simulink model "six_rod_tensegrity_model_2021a"  (R2021a)
settings: Solver=ode45  StartTime=0  StopTime=Inf  RelTol=1e-1
values from neighbouring files (symbols this model uses):
  grivity_z = -9.80665    [code_for_6_rods_tensegrity.m]
  i = 19    [drive_params.m]
  Jsum = Jd + Jp + Jnagr    (= 9.27e-08)    [drive_params.m]
  km = 9.32 / 1000    (= 0.00932)    [drive_params.m]
  kpdr = 0.81    [drive_params.m]
  kw = 60 / (2*pi * 1020)    (= 0.00936205547599)    [drive_params.m]
  L = 0.14 / 1000    (= 0.00014)    [drive_params.m]
  load_mass = 0.5    [code_for_6_rods_tensegrity.m]
  plane_offset = -(rod_length/2 + 0.032 + rod_radius)    [code_for_6_rods_tensegrity.m]
  R = 5.3    [drive_params.m]
  rod_end_drive_offset = spool_active_length    (= 0.015)    [code_for_6_rods_tensegrity.m]
  rod_end_mass = 0.05    [code_for_6_rods_tensegrity.m]
  rod_end_mass_with_drive = 0.2    [code_for_6_rods_tensegrity.m]
  rod_mass = 0.028    [code_for_6_rods_tensegrity.m]
  rod_mass_with_drive = 0.038    [code_for_6_rods_tensegrity.m]
  rod_radius = 0.004    [code_for_6_rods_tensegrity.m]
undefined symbols (not defined in the file or in its folder): Left_end_cap_1_1, Left_end_cap_2_3, Left_end_cap_3_5, Left_end_cap_4_7, Left_end_cap_5_9, Left_end_cap_6_11, Right_end_cap_1_2, Right_end_cap_2_4, Right_end_cap_3_6, Right_end_cap_4_8, Right_end_cap_5_10, Right_end_cap_6_12, Rod_center_1, Rod_center_2, Rod_center_3, Rod_center_4, Rod_center_5, Rod_center_6, sigbuilder_block, X, Y, Z
libraries: sm_lib x403, nesl_utility x73
(part 4 of 5)

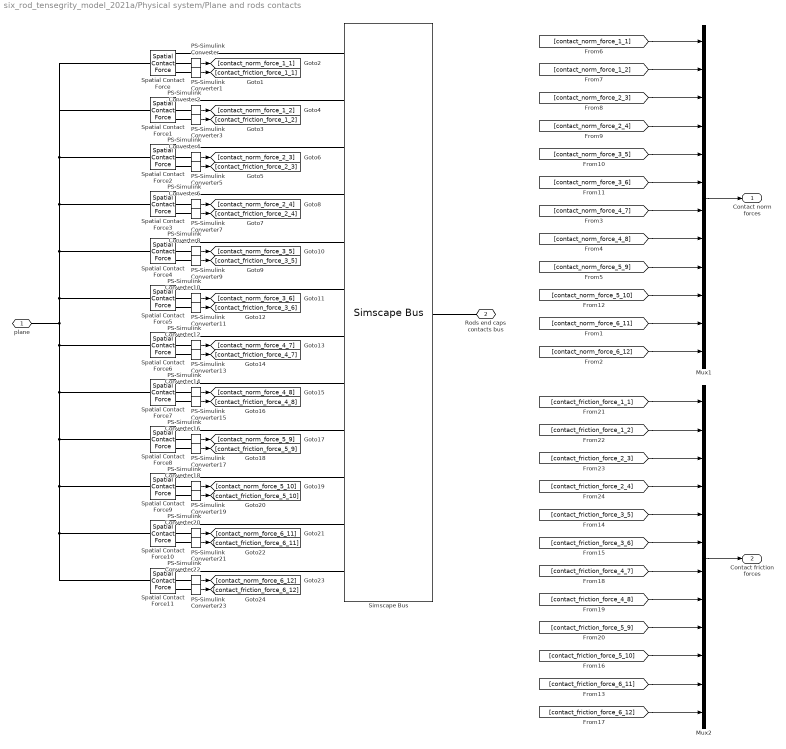
== system six_rod_tensegrity_model_2021a/Physical system/Plane and rods contacts ==
  Mux1 : Mux  Inputs=12
  Mux2 : Mux  Inputs=12
  PS-Simulink Converter{,1..23} (24 alike) : nesl_utility/PS-Simulink Converter  PhysicalDomain=network_engine_domain  SubClassName=ps_output  LeftPortType=input  RightPortType=output  PseudoPeriodic=off  Frequencies=[]  Unit=N  AffineConversion=off
      settings: SourceProductBaseCode=PW,SS
  Simscape Bus : SimscapeBus  HierarchyStrings=Left_end_cap_contact_1_1;Right_end_cap_contact_1_2;Left_end_cap_contact_2_3;Right_end_cap_contact_2_4;Left_end_cap_contact_3_5;Right_end_cap_contact_3_6;Left_end_cap_contact_4_7;Right_end_cap_contact_4_8;Left_end_cap_contact_5_9;Right_end_cap_contact_5_10;Left_end_cap_contact_6_11;Right_end_cap_contact_6_12
  Spatial Contact Force{,1..11} (12 alike) : sm_lib/Forces and Torques/Spatial Contact Force  CoefficientOfDynamicFriction=contact_dynamic_friction_coef  CoefficientOfStaticFriction=contact_static_friction_coef  SenseContactBaseRotation=off  SenseContactBaseTranslation=off  NormalDamping=contact_damping  NormalDampingUnits=N/(m/s)  SenseContactFollowerRotation=off  SenseContactFollowerTranslation=off  SenseContactSignal=off  NormalStiffness=contact_stiffness  NormalStiffnessUnits=N/m  FrictionalCriticalVelocity=contact_critical_velocity  FrictionalCriticalVelocityUnits=m/s  ZeroCrossDetectContactStartAndEnd=off  FrictionType=SmoothStickSlip  SenseFrictionalForceMagnitude=on  SenseNormalForceMagnitude=on  NormalForceType=SmoothSpringDamper  SenseNormalVelocity=off  SenseSeparationDistance=off  SenseTangentialVelocity=off  SenseTangentialVelocityMagnitude=off  NormalTransitionRegionWidth=contact_transition_region_width  NormalTransitionRegionWidthUnits=m
  plane : PMIOPort  Side=Left
  Rods end caps contacts bus : PMIOPort  Port=2  Side=Right
  Contact norm forces : Outport
  Contact friction forces : Outport  Port=2
  wires:
  PS-Simulink Converter/1 -> [contact_norm_force_1_1]
  PS-Simulink Converter1/1 -> [contact_friction_force_1_1]
  PS-Simulink Converter2/1 -> [contact_norm_force_1_2]
  PS-Simulink Converter3/1 -> [contact_friction_force_1_2]
  PS-Simulink Converter5/1 -> [contact_friction_force_2_3]
  PS-Simulink Converter4/1 -> [contact_norm_force_2_3]
  PS-Simulink Converter6/1 -> [contact_norm_force_2_4]
  PS-Simulink Converter7/1 -> [contact_friction_force_2_4]
  PS-Simulink Converter9/1 -> [contact_friction_force_3_5]
  PS-Simulink Converter8/1 -> [contact_norm_force_3_5]
  PS-Simulink Converter10/1 -> [contact_norm_force_3_6]
  PS-Simulink Converter11/1 -> [contact_friction_force_3_6]
  PS-Simulink Converter13/1 -> [contact_friction_force_4_7]
  PS-Simulink Converter12/1 -> [contact_norm_force_4_7]
  PS-Simulink Converter14/1 -> [contact_norm_force_4_8]
  PS-Simulink Converter15/1 -> [contact_friction_force_4_8]
  PS-Simulink Converter17/1 -> [contact_friction_force_5_9]
  PS-Simulink Converter16/1 -> [contact_norm_force_5_9]
  PS-Simulink Converter18/1 -> [contact_norm_force_5_10]
  PS-Simulink Converter19/1 -> [contact_friction_force_5_10]
  PS-Simulink Converter21/1 -> [contact_friction_force_6_11]
  PS-Simulink Converter20/1 -> [contact_norm_force_6_11]
  PS-Simulink Converter22/1 -> [contact_norm_force_6_12]
  PS-Simulink Converter23/1 -> [contact_friction_force_6_12]
  [contact_norm_force_1_1] -> Mux1/1
  [contact_norm_force_2_3] -> Mux1/3
  [contact_norm_force_3_6] -> Mux1/6
  [contact_norm_force_2_4] -> Mux1/4
  Mux1/1 -> Contact norm forces/1
  [contact_norm_force_1_2] -> Mux1/2
  [contact_norm_force_3_5] -> Mux1/5
  [contact_norm_force_4_7] -> Mux1/7
  [contact_norm_force_4_8] -> Mux1/8
  [contact_norm_force_5_9] -> Mux1/9
  [contact_norm_force_5_10] -> Mux1/10
  [contact_norm_force_6_11] -> Mux1/11
  [contact_norm_force_6_12] -> Mux1/12
  [contact_friction_force_6_12] -> Mux2/12
  [contact_friction_force_6_11] -> Mux2/11
  [contact_friction_force_5_10] -> Mux2/10
  [contact_friction_force_5_9] -> Mux2/9
  [contact_friction_force_4_8] -> Mux2/8
  [contact_friction_force_4_7] -> Mux2/7
  [contact_friction_force_3_5] -> Mux2/5
  [contact_friction_force_1_2] -> Mux2/2
  Mux2/1 -> Contact friction forces/1
  [contact_friction_force_2_4] -> Mux2/4
  [contact_friction_force_3_6] -> Mux2/6
  [contact_friction_force_2_3] -> Mux2/3
  [contact_friction_force_1_1] -> Mux2/1
  connections:
  Spatial Contact Force1/RConn1 -- Simscape Bus/LConn2
  Spatial Contact Force3/RConn1 -- Simscape Bus/LConn4
  Spatial Contact Force2/RConn1 -- Simscape Bus/LConn3
  Spatial Contact Force4/RConn1 -- Simscape Bus/LConn5
  Spatial Contact Force5/RConn1 -- Simscape Bus/LConn6
  Spatial Contact Force4/LConn1 -- Spatial Contact Force3/LConn1 -- Spatial Contact Force2/LConn1 -- Spatial Contact Force1/LConn1 -- Spatial Contact Force/LConn1 -- Spatial Contact Force5/LConn1 -- plane/RConn1 -- Spatial Contact Force6/LConn1 -- Spatial Contact Force7/LConn1 -- Spatial Contact Force8/LConn1 -- Spatial Contact Force9/LConn1 -- Spatial Contact Force11/LConn1 -- Spatial Contact Force10/LConn1
  Spatial Contact Force6/RConn1 -- Simscape Bus/LConn7
  Spatial Contact Force11/RConn1 -- Simscape Bus/LConn12
  Spatial Contact Force8/RConn1 -- Simscape Bus/LConn9
  Spatial Contact Force7/RConn1 -- Simscape Bus/LConn8
  Spatial Contact Force10/RConn1 -- Simscape Bus/LConn11
  Spatial Contact Force/RConn1 -- Simscape Bus/LConn1
  Spatial Contact Force9/RConn1 -- Simscape Bus/LConn10
  Rods end caps contacts bus/RConn1 -- Simscape Bus/RConn1
  PS-Simulink Converter/LConn1 -- Spatial Contact Force/RConn2
  Spatial Contact Force/RConn3 -- PS-Simulink Converter1/LConn1
  Spatial Contact Force1/RConn2 -- PS-Simulink Converter2/LConn1
  Spatial Contact Force1/RConn3 -- PS-Simulink Converter3/LConn1
  Spatial Contact Force2/RConn3 -- PS-Simulink Converter5/LConn1
  Spatial Contact Force2/RConn2 -- PS-Simulink Converter4/LConn1
  Spatial Contact Force3/RConn2 -- PS-Simulink Converter6/LConn1
  Spatial Contact Force3/RConn3 -- PS-Simulink Converter7/LConn1
  Spatial Contact Force4/RConn2 -- PS-Simulink Converter8/LConn1
  Spatial Contact Force4/RConn3 -- PS-Simulink Converter9/LConn1
  Spatial Contact Force5/RConn3 -- PS-Simulink Converter11/LConn1
  Spatial Contact Force5/RConn2 -- PS-Simulink Converter10/LConn1
  Spatial Contact Force6/RConn3 -- PS-Simulink Converter13/LConn1
  Spatial Contact Force6/RConn2 -- PS-Simulink Converter12/LConn1
  Spatial Contact Force10/RConn2 -- PS-Simulink Converter20/LConn1
  Spatial Contact Force10/RConn3 -- PS-Simulink Converter21/LConn1
  Spatial Contact Force9/RConn3 -- PS-Simulink Converter19/LConn1
  Spatial Contact Force9/RConn2 -- PS-Simulink Converter18/LConn1
  Spatial Contact Force8/RConn3 -- PS-Simulink Converter17/LConn1
  Spatial Contact Force8/RConn2 -- PS-Simulink Converter16/LConn1
  Spatial Contact Force7/RConn3 -- PS-Simulink Converter15/LConn1
  Spatial Contact Force7/RConn2 -- PS-Simulink Converter14/LConn1
  Spatial Contact Force11/RConn3 -- PS-Simulink Converter23/LConn1
  Spatial Contact Force11/RConn2 -- PS-Simulink Converter22/LConn1

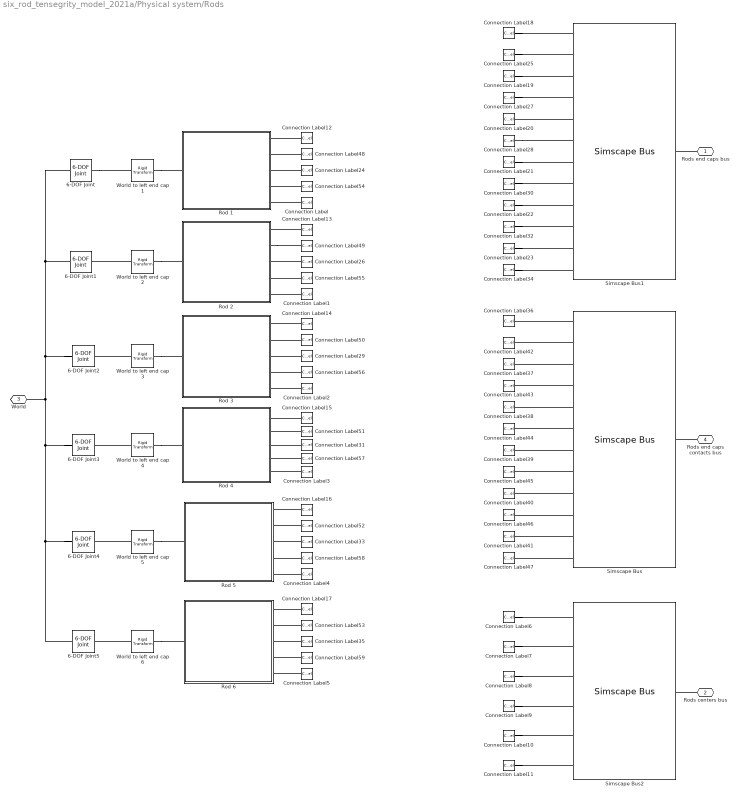
== system six_rod_tensegrity_model_2021a/Physical system/Rods ==
  6-DOF Joint{,1..5} (6 alike) : sm_lib/Joints/6-DOF Joint  JointMode=Normal  SenseConstraintForce=off  SenseConstraintForceX=off  SenseConstraintForceY=off  SenseConstraintForceZ=off  SenseConstraintTorque=off  SenseConstraintTorqueX=off  SenseConstraintTorqueY=off  SenseConstraintTorqueZ=off  SenseTotalForce=off  SenseTotalForceX=off  SenseTotalForceY=off  SenseTotalForceZ=off  SenseTotalTorque=off  SenseTotalTorqueX=off  SenseTotalTorqueY=off  SenseTotalTorqueZ=off  CompositeWrenchDir=FollowerOnBase  CompositeWrenchFrame=BaseFrame  PxEquilibriumPosition=0  PxEquilibriumPositionUnits=m  PxSpringStiffness=0  PxSpringStiffnessUnits=N/m  PxDampingCoefficient=0  PxDampingCoefficientUnits=N/(m/s)  PxTorqueActuationMode=NoTorque  PxMotionActuationMode=ComputedMotion  PxSensePosition=off  PxSenseVelocity=off  PxSenseAcceleration=off  PxSenseTorqueForce=off  PxSenseLowerLimitTorqueForce=off  PxSenseUpperLimitTorqueForce=off  PxLowerLimitSpecify=off  PxLowerLimitBound=-1  PxLowerLimitBoundUnits=m  PxLowerLimitStiffness=1e6  PxLowerLimitStiffnessUnits=N/m  PxLowerLimitDamping=1e3  PxLowerLimitDampingUnits=N/(m/s)  PxLowerLimitTransitionRegionWidth=1e-4  PxLowerLimitTransitionRegionWidthUnits=m  PxUpperLimitSpecify=off  PxUpperLimitBound=1  PxUpperLimitBoundUnits=m  PxUpperLimitStiffness=1e6  PxUpperLimitStiffnessUnits=N/m  PxUpperLimitDamping=1e3  PxUpperLimitDampingUnits=N/(m/s)  PxUpperLimitTransitionRegionWidth=1e-4  PxUpperLimitTransitionRegionWidthUnits=m  PxPositionTargetSpecify=off  PxPositionTargetPriority=High  PxPositionTargetValue=0  PxPositionTargetValueUnits=m  PxVelocityTargetSpecify=off  PxVelocityTargetPriority=High  PxVelocityTargetValue=0  PxVelocityTargetValueUnits=m/s  PyEquilibriumPosition=0  PyEquilibriumPositionUnits=m  PySpringStiffness=0  PySpringStiffnessUnits=N/m  PyDampingCoefficient=0  PyDampingCoefficientUnits=N/(m/s)  PyTorqueActuationMode=NoTorque  PyMotionActuationMode=ComputedMotion  PySensePosition=off  PySenseVelocity=off  PySenseAcceleration=off  PySenseTorqueForce=off  PySenseLowerLimitTorqueForce=off  PySenseUpperLimitTorqueForce=off  PyLowerLimitSpecify=off  PyLowerLimitBound=-1  PyLowerLimitBoundUnits=m  PyLowerLimitStiffness=1e6  PyLowerLimitStiffnessUnits=N/m  PyLowerLimitDamping=1e3  PyLowerLimitDampingUnits=N/(m/s)  PyLowerLimitTransitionRegionWidth=1e-4  PyLowerLimitTransitionRegionWidthUnits=m  PyUpperLimitSpecify=off  PyUpperLimitBound=1  PyUpperLimitBoundUnits=m  PyUpperLimitStiffness=1e6  PyUpperLimitStiffnessUnits=N/m  PyUpperLimitDamping=1e3  PyUpperLimitDampingUnits=N/(m/s)  PyUpperLimitTransitionRegionWidth=1e-4  PyUpperLimitTransitionRegionWidthUnits=m  PyPositionTargetSpecify=off  PyPositionTargetPriority=High  PyPositionTargetValue=0  PyPositionTargetValueUnits=m  PyVelocityTargetSpecify=off  PyVelocityTargetPriority=High  PyVelocityTargetValue=0  PyVelocityTargetValueUnits=m/s  PzEquilibriumPosition=0  PzEquilibriumPositionUnits=m  PzSpringStiffness=0  PzSpringStiffnessUnits=N/m  PzDampingCoefficient=0  PzDampingCoefficientUnits=N/(m/s)  PzTorqueActuationMode=NoTorque  PzMotionActuationMode=ComputedMotion  PzSensePosition=off  PzSenseVelocity=off  PzSenseAcceleration=off  PzSenseTorqueForce=off  PzSenseLowerLimitTorqueForce=off  PzSenseUpperLimitTorqueForce=off  PzLowerLimitSpecify=off  PzLowerLimitBound=-1  PzLowerLimitBoundUnits=m  PzLowerLimitStiffness=1e6  PzLowerLimitStiffnessUnits=N/m  PzLowerLimitDamping=1e3  PzLowerLimitDampingUnits=N/(m/s)  PzLowerLimitTransitionRegionWidth=1e-4  PzLowerLimitTransitionRegionWidthUnits=m  PzUpperLimitSpecify=off  PzUpperLimitBound=1  PzUpperLimitBoundUnits=m  PzUpperLimitStiffness=1e6  PzUpperLimitStiffnessUnits=N/m  PzUpperLimitDamping=1e3  PzUpperLimitDampingUnits=N/(m/s)  PzUpperLimitTransitionRegionWidth=1e-4  PzUpperLimitTransitionRegionWidthUnits=m  PzPositionTargetSpecify=off  PzPositionTargetPriority=High  PzPositionTargetValue=0  PzPositionTargetValueUnits=m  PzVelocityTargetSpecify=off  PzVelocityTargetPriority=High  PzVelocityTargetValue=0  PzVelocityTargetValueUnits=m/s  SphDefPosRotationMethod=None  SphDefPosRotationAngleUnits=deg  SphDefPosRotationStandardAxis=+Z  SphDefPosRotationAngle=0.0  SphDefPosRotationArbitraryAxis=[0 0 1]  SphDefPosFollAlignAxisA=+X  SphDefPosBaseAlignAxisA=+Y  SphDefPosFollAlignAxisB=+Y  SphDefPosBaseAlignAxisB=+Z  SphDefPosRotationSequenceAxes=FollowerAxes  SphDefPosRotationSequence=XYX  SphDefPosRotationSequenceAngles=[0 0 0]  SphDefPosRotationSequenceAnglesUnits=deg  SphDefPosRotationMatrix=[1 0 0; 0 1 0; 0 0 1]  SphEqPosRotationMethod=None  SphEqPosRotationAngleUnits=deg  SphEqPosRotationStandardAxis=+Z  SphEqPosRotationAngle=0.0  SphEqPosRotationArbitraryAxis=[0 0 1]  SphEqPosFollAlignAxisA=+X  SphEqPosBaseAlignAxisA=+Y  SphEqPosFollAlignAxisB=+Y  SphEqPosBaseAlignAxisB=+Z  SphEqPosRotationSequenceAxes=FollowerAxes  SphEqPosRotationSequence=XYX  SphEqPosRotationSequenceAngles=[0 0 0]  SphEqPosRotationSequenceAnglesUnits=deg  SphEqPosRotationMatrix=[1 0 0; 0 1 0; 0 0 1]  SphSpringStiffness=0  SphSpringStiffnessUnits=N*m/deg  SphDampingCoefficient=0  SphDampingCoefficientUnits=N*m/(deg/s)  SphActuateTorqueX=off  SphActuateTorqueY=off  SphActuateTorqueZ=off  SphActuateTorque=off  SphTorqueActuationMode=NoTorque  SphMotionActuationMode=ComputedMotion  SphActuationFrame=BaseFrame  SphSensePosition=off  SphSenseVelocityX=off  SphSenseVelocityY=off  SphSenseVelocityZ=off  SphSenseVelocity=off  SphSenseAccelerationX=off  SphSenseAccelerationY=off  SphSenseAccelerationZ=off  SphSenseAcceleration=off  SphSenseTorqueX=off  SphSenseTorqueY=off  SphSenseTorqueZ=off  SphSenseTorqueForce=off  SphSenseLowerLimitTorqueMag=off  SphSenseUpperLimitTorqueMag=off  SphSensingFrame=BaseFrame  SphLowerLimitSpecify=off  SphLowerLimitBound=15  SphLowerLimitBoundUnits=deg  SphLowerLimitStiffness=1e4  SphLowerLimitStiffnessUnits=N*m/deg  SphLowerLimitDamping=10  SphLowerLimitDampingUnits=N*m/(deg/s)  SphLowerLimitTransitionRegionWidth=0.1  SphLowerLimitTransitionRegionWidthUnits=deg  SphUpperLimitSpecify=off  SphUpperLimitBound=45  SphUpperLimitBoundUnits=deg  SphUpperLimitStiffness=1e4  SphUpperLimitStiffnessUnits=N*m/deg  SphUpperLimitDamping=10  SphUpperLimitDampingUnits=N*m/(deg/s)  SphUpperLimitTransitionRegionWidth=0.1  SphUpperLimitTransitionRegionWidthUnits=deg  SphPositionTargetRotationMethod=None  SphPositionTargetRotationAngleUnits=deg  SphPositionTargetRotationStandardAxis=+Z  SphPositionTargetRotationAngle=0.0  SphPositionTargetRotationArbitraryAxis=[0 0 1]  SphPositionTargetFollAlignAxisA=+X  SphPositionTargetBaseAlignAxisA=+Y  SphPositionTargetFollAlignAxisB=+Y  SphPositionTargetBaseAlignAxisB=+Z  SphPositionTargetRotationSequenceAxes=FollowerAxes  SphPositionTargetRotationSequence=XYX  SphPositionTargetRotationSequenceAngles=[0 0 0]  SphPositionTargetRotationSequenceAnglesUnits=deg  SphPositionTargetRotationMatrix=[1 0 0; 0 1 0; 0 0 1]  SphPositionTargetSpecify=off  SphPositionTargetPriority=High  SphVelocityTargetValue=[0 0 0]  SphVelocityTargetValueUnits=deg/s  SphVelocityTargetSpecify=off  SphVelocityTargetPriority=High  SphVelocityTargetInFollowerFrame=on
  Connection Label : ConnectionLabel  Label=Rod_center_1
  Connection Label1 : ConnectionLabel  Label=Rod_center_2
  Connection Label10 : ConnectionLabel  Label=Rod_center_5
  Connection Label11 : ConnectionLabel  Label=Rod_center_6
  Connection Label12 : ConnectionLabel  Label=Left_end_cap_1_1
  Connection Label13 : ConnectionLabel  Label=Left_end_cap_2_3
  Connection Label14 : ConnectionLabel  Label=Left_end_cap_3_5
  Connection Label15 : ConnectionLabel  Label=Left_end_cap_4_7
  Connection Label16 : ConnectionLabel  Label=Left_end_cap_5_9
  Connection Label17 : ConnectionLabel  Label=Left_end_cap_6_11
  Connection Label18 : ConnectionLabel  Label=Left_end_cap_1_1
  Connection Label19 : ConnectionLabel  Label=Left_end_cap_2_3
  Connection Label2 : ConnectionLabel  Label=Rod_center_3
  Connection Label20 : ConnectionLabel  Label=Left_end_cap_3_5
  Connection Label21 : ConnectionLabel  Label=Left_end_cap_4_7
  Connection Label22 : ConnectionLabel  Label=Left_end_cap_5_9
  Connection Label23 : ConnectionLabel  Label=Left_end_cap_6_11
  Connection Label24 : ConnectionLabel  Label=Right_end_cap_1_2
  Connection Label25 : ConnectionLabel  Label=Right_end_cap_1_2
  Connection Label26 : ConnectionLabel  Label=Right_end_cap_2_4
  Connection Label27 : ConnectionLabel  Label=Right_end_cap_2_4
  Connection Label28 : ConnectionLabel  Label=Right_end_cap_3_6
  Connection Label29 : ConnectionLabel  Label=Right_end_cap_3_6
  Connection Label3 : ConnectionLabel  Label=Rod_center_4
  Connection Label30 : ConnectionLabel  Label=Right_end_cap_4_8
  Connection Label31 : ConnectionLabel  Label=Right_end_cap_4_8
  Connection Label32 : ConnectionLabel  Label=Right_end_cap_5_10
  Connection Label33 : ConnectionLabel  Label=Right_end_cap_5_10
  Connection Label34 : ConnectionLabel  Label=Right_end_cap_6_12
  Connection Label35 : ConnectionLabel  Label=Right_end_cap_6_12
  Connection Label36 : ConnectionLabel  Label=Left_end_cap_contact_1_1
  Connection Label37 : ConnectionLabel  Label=Left_end_cap_contact_2_3
  Connection Label38 : ConnectionLabel  Label=Left_end_cap_contact_3_5
  Connection Label39 : ConnectionLabel  Label=Left_end_cap_contact_4_7
  Connection Label4 : ConnectionLabel  Label=Rod_center_5
  Connection Label40 : ConnectionLabel  Label=Left_end_cap_contact_5_9
  Connection Label41 : ConnectionLabel  Label=Left_end_cap_contact_6_11
  Connection Label42 : ConnectionLabel  Label=Right_end_cap_contact_1_2
  Connection Label43 : ConnectionLabel  Label=Right_end_cap_contact_2_4
  Connection Label44 : ConnectionLabel  Label=Right_end_cap_contact_3_6
  Connection Label45 : ConnectionLabel  Label=Right_end_cap_contact_4_8
  Connection Label46 : ConnectionLabel  Label=Right_end_cap_contact_5_10
  Connection Label47 : ConnectionLabel  Label=Right_end_cap_contact_6_12
  Connection Label48 : ConnectionLabel  Label=Left_end_cap_contact_1_1
  Connection Label49 : ConnectionLabel  Label=Left_end_cap_contact_2_3
  Connection Label5 : ConnectionLabel  Label=Rod_center_6
  Connection Label50 : ConnectionLabel  Label=Left_end_cap_contact_3_5
  Connection Label51 : ConnectionLabel  Label=Left_end_cap_contact_4_7
  Connection Label52 : ConnectionLabel  Label=Left_end_cap_contact_5_9
  Connection Label53 : ConnectionLabel  Label=Left_end_cap_contact_6_11
  Connection Label54 : ConnectionLabel  Label=Right_end_cap_contact_1_2
  Connection Label55 : ConnectionLabel  Label=Right_end_cap_contact_2_4
  Connection Label56 : ConnectionLabel  Label=Right_end_cap_contact_3_6
  Connection Label57 : ConnectionLabel  Label=Right_end_cap_contact_4_8
  Connection Label58 : ConnectionLabel  Label=Right_end_cap_contact_5_10
  Connection Label59 : ConnectionLabel  Label=Right_end_cap_contact_6_12
  Connection Label6 : ConnectionLabel  Label=Rod_center_1
  Connection Label7 : ConnectionLabel  Label=Rod_center_2
  Connection Label8 : ConnectionLabel  Label=Rod_center_3
  Connection Label9 : ConnectionLabel  Label=Rod_center_4
  Rod 1 : Subsystem
      mask Display: image(imread('tensegrity_rod.jpg'))
  Rod 2 : Subsystem
      mask Display: image(imread('tensegrity_rod.jpg'))
  Rod 3 : Subsystem
      mask Display: image(imread('tensegrity_rod.jpg'))
  Rod 4 : Subsystem
      mask Display: image(imread('tensegrity_rod.jpg'))
  Rod 5 : Subsystem
      mask Display: image(imread('tensegrity_rod.jpg'))
  Rod 6 : Subsystem
      mask Display: image(imread('tensegrity_rod.jpg'))
  Simscape Bus : SimscapeBus  HierarchyStrings=Left_end_cap_contact_1_1;Right_end_cap_contact_1_2;Left_end_cap_contact_2_3;Right_end_cap_contact_2_4;Left_end_cap_contact_3_5;Right_end_cap_contact_3_6;Left_end_cap_contact_4_7;Right_end_cap_contact_4_8;Left_end_cap_contact_5_9;Right_end_cap_contact_5_10;Left_end_cap_contact_6_11;Right_end_cap_contact_6_12
  Simscape Bus1 : SimscapeBus  HierarchyStrings=Left_end_cap_1_1;Right_end_cap_1_2;Left_end_cap_2_3;Right_end_cap_2_4;Left_end_cap_3_5;Right_end_cap_3_6;Left_end_cap_4_7;Right_end_cap_4_8;Left_end_cap_5_9;Right_end_cap_5_10;Left_end_cap_6_11;Right_end_cap_6_12
  Simscape Bus2 : SimscapeBus  HierarchyStrings=Rod_center_1;Rod_center_2;Rod_center_3;Rod_center_4;Rod_center_5;Rod_center_6
  World to left end cap 1 : sm_lib/Frames and Transforms/Rigid Transform  TranslationMethod=Cartesian  TranslationStandardOffset=250  TranslationLengthUnit=m  TranslationStandardAxis=+Z  TranslationCartesianOffset=rod_start_point_1  TranslationROffset=0  TranslationROffsetUnits=m  TranslationZOffset=0  TranslationZOffsetUnits=m  TranslationThetaOffset=0  TranslationThetaOffsetUnits=deg  RotationMethod=ArbitraryAxis  RotationAngleUnits=deg  RotationStandardAxis=+Y  RotationAngle=rod_angle_1  RotationArbitraryAxis=rod_rotation_axis_1  FollAlignAxisA=+Z  BaseAlignAxisA=+X  FollAlignAxisB=+Y  BaseAlignAxisB=+Z  RotationSequenceAxes=BaseAxes  RotationSequence=YZX  RotationSequenceAngles=[90 63.43 0]  RotationSequenceAnglesUnits=deg  RotationMatrix=[1 0 0; 0 1 0; 0 0 1]
  World to left end cap 2 : sm_lib/Frames and Transforms/Rigid Transform  TranslationMethod=Cartesian  TranslationStandardOffset=250  TranslationLengthUnit=m  TranslationStandardAxis=+Z  TranslationCartesianOffset=rod_start_point_2  TranslationROffset=0  TranslationROffsetUnits=m  TranslationZOffset=0  TranslationZOffsetUnits=m  TranslationThetaOffset=0  TranslationThetaOffsetUnits=deg  RotationMethod=ArbitraryAxis  RotationAngleUnits=deg  RotationStandardAxis=+Y  RotationAngle=rod_angle_2  RotationArbitraryAxis=rod_rotation_axis_2  FollAlignAxisA=+Z  BaseAlignAxisA=+X  FollAlignAxisB=+Y  BaseAlignAxisB=+Z  RotationSequenceAxes=BaseAxes  RotationSequence=YZX  RotationSequenceAngles=[90 63.43 0]  RotationSequenceAnglesUnits=deg  RotationMatrix=[1 0 0; 0 1 0; 0 0 1]
  World to left end cap 3 : sm_lib/Frames and Transforms/Rigid Transform  TranslationMethod=Cartesian  TranslationStandardOffset=250  TranslationLengthUnit=m  TranslationStandardAxis=+Z  TranslationCartesianOffset=rod_start_point_3  TranslationROffset=0  TranslationROffsetUnits=m  TranslationZOffset=0  TranslationZOffsetUnits=m  TranslationThetaOffset=0  TranslationThetaOffsetUnits=deg  RotationMethod=ArbitraryAxis  RotationAngleUnits=deg  RotationStandardAxis=+Y  RotationAngle=rod_angle_3  RotationArbitraryAxis=rod_rotation_axis_3  FollAlignAxisA=+Z  BaseAlignAxisA=+X  FollAlignAxisB=+Y  BaseAlignAxisB=+Z  RotationSequenceAxes=BaseAxes  RotationSequence=YZX  RotationSequenceAngles=[90 63.43 0]  RotationSequenceAnglesUnits=deg  RotationMatrix=[1 0 0; 0 1 0; 0 0 1]
  World to left end cap 4 : sm_lib/Frames and Transforms/Rigid Transform  TranslationMethod=Cartesian  TranslationStandardOffset=250  TranslationLengthUnit=m  TranslationStandardAxis=+Z  TranslationCartesianOffset=rod_start_point_4  TranslationROffset=0  TranslationROffsetUnits=m  TranslationZOffset=0  TranslationZOffsetUnits=m  TranslationThetaOffset=0  TranslationThetaOffsetUnits=deg  RotationMethod=ArbitraryAxis  RotationAngleUnits=deg  RotationStandardAxis=+Y  RotationAngle=rod_angle_4  RotationArbitraryAxis=rod_rotation_axis_4  FollAlignAxisA=+Z  BaseAlignAxisA=+X  FollAlignAxisB=+Y  BaseAlignAxisB=+Z  RotationSequenceAxes=BaseAxes  RotationSequence=YZX  RotationSequenceAngles=[90 63.43 0]  RotationSequenceAnglesUnits=deg  RotationMatrix=[1 0 0; 0 1 0; 0 0 1]
  World to left end cap 5 : sm_lib/Frames and Transforms/Rigid Transform  TranslationMethod=Cartesian  TranslationStandardOffset=250  TranslationLengthUnit=m  TranslationStandardAxis=+Z  TranslationCartesianOffset=rod_start_point_5  TranslationROffset=0  TranslationROffsetUnits=m  TranslationZOffset=0  TranslationZOffsetUnits=m  TranslationThetaOffset=0  TranslationThetaOffsetUnits=deg  RotationMethod=ArbitraryAxis  RotationAngleUnits=deg  RotationStandardAxis=+Y  RotationAngle=rod_angle_5  RotationArbitraryAxis=rod_rotation_axis_5  FollAlignAxisA=+Z  BaseAlignAxisA=+X  FollAlignAxisB=+Y  BaseAlignAxisB=+Z  RotationSequenceAxes=BaseAxes  RotationSequence=YZX  RotationSequenceAngles=[90 63.43 0]  RotationSequenceAnglesUnits=deg  RotationMatrix=[1 0 0; 0 1 0; 0 0 1]
  World to left end cap 6 : sm_lib/Frames and Transforms/Rigid Transform  TranslationMethod=Cartesian  TranslationStandardOffset=250  TranslationLengthUnit=m  TranslationStandardAxis=+Z  TranslationCartesianOffset=rod_start_point_6  TranslationROffset=0  TranslationROffsetUnits=m  TranslationZOffset=0  TranslationZOffsetUnits=m  TranslationThetaOffset=0  TranslationThetaOffsetUnits=deg  RotationMethod=ArbitraryAxis  RotationAngleUnits=deg  RotationStandardAxis=+Y  RotationAngle=rod_angle_6  RotationArbitraryAxis=rod_rotation_axis_6  FollAlignAxisA=+Z  BaseAlignAxisA=+X  FollAlignAxisB=+Y  BaseAlignAxisB=+Z  RotationSequenceAxes=BaseAxes  RotationSequence=YZX  RotationSequenceAngles=[90 63.43 0]  RotationSequenceAnglesUnits=deg  RotationMatrix=[1 0 0; 0 1 0; 0 0 1]
  Rods end caps bus : PMIOPort  Side=Left
  Rods centers bus : PMIOPort  Port=2  Side=Left
  World : PMIOPort  Port=3  Side=Left
  Rods end caps contacts bus : PMIOPort  Port=4  Side=Right
  connections:
  6-DOF Joint/RConn1 -- World to left end cap 1/LConn1
  6-DOF Joint5/LConn1 -- 6-DOF Joint4/LConn1 -- 6-DOF Joint3/LConn1 -- 6-DOF Joint2/LConn1 -- 6-DOF Joint1/LConn1 -- 6-DOF Joint/LConn1 -- World/RConn1
  World to left end cap 2/RConn1 -- Rod 2/LConn1
  World to left end cap 5/LConn1 -- 6-DOF Joint4/RConn1
  World to left end cap 1/RConn1 -- Rod 1/LConn1
  World to left end cap 2/LConn1 -- 6-DOF Joint1/RConn1
  World to left end cap 6/LConn1 -- 6-DOF Joint5/RConn1
  World to left end cap 3/RConn1 -- Rod 3/LConn1
  World to left end cap 3/LConn1 -- 6-DOF Joint2/RConn1
  World to left end cap 6/RConn1 -- Rod 6/LConn1
  World to left end cap 4/LConn1 -- 6-DOF Joint3/RConn1
  World to left end cap 5/RConn1 -- Rod 5/LConn1
  World to left end cap 4/RConn1 -- Rod 4/LConn1
  Rods end caps contacts bus/RConn1 -- Simscape Bus/RConn1
  Rods end caps bus/RConn1 -- Simscape Bus1/RConn1
  Rods centers bus/RConn1 -- Simscape Bus2/RConn1
  Connection Label11/LConn1 -- Simscape Bus2/LConn6
  Connection Label10/LConn1 -- Simscape Bus2/LConn5
  Connection Label9/LConn1 -- Simscape Bus2/LConn4
  Connection Label8/LConn1 -- Simscape Bus2/LConn3
  Connection Label7/LConn1 -- Simscape Bus2/LConn2
  Connection Label6/LConn1 -- Simscape Bus2/LConn1
  Connection Label/LConn1 -- Rod 1/RConn5
  Connection Label1/LConn1 -- Rod 2/RConn5
  Connection Label2/LConn1 -- Rod 3/RConn5
  Connection Label3/LConn1 -- Rod 4/RConn5
  Connection Label4/LConn1 -- Rod 5/RConn5
  Connection Label5/LConn1 -- Rod 6/RConn5
  Connection Label12/LConn1 -- Rod 1/RConn1
  Connection Label13/LConn1 -- Rod 2/RConn1
  Connection Label14/LConn1 -- Rod 3/RConn1
  Connection Label15/LConn1 -- Rod 4/RConn1
  Connection Label16/LConn1 -- Rod 5/RConn1
  Connection Label17/LConn1 -- Rod 6/RConn1
  Connection Label18/LConn1 -- Simscape Bus1/LConn1
  Connection Label19/LConn1 -- Simscape Bus1/LConn3
  Simscape Bus1/LConn5 -- Connection Label20/LConn1
  Connection Label21/LConn1 -- Simscape Bus1/LConn7
  Connection Label22/LConn1 -- Simscape Bus1/LConn9
  Connection Label23/LConn1 -- Simscape Bus1/LConn11
  Connection Label24/LConn1 -- Rod 1/RConn3
  Connection Label25/LConn1 -- Simscape Bus1/LConn2
  Connection Label26/LConn1 -- Rod 2/RConn3
  Connection Label27/LConn1 -- Simscape Bus1/LConn4
  Connection Label29/LConn1 -- Rod 3/RConn3
  Connection Label30/LConn1 -- Simscape Bus1/LConn8
  Connection Label31/LConn1 -- Rod 4/RConn3
  Connection Label32/LConn1 -- Simscape Bus1/LConn10
  Connection Label33/LConn1 -- Rod 5/RConn3
  Connection Label34/LConn1 -- Simscape Bus1/LConn12
  Connection Label35/LConn1 -- Rod 6/RConn3
  Simscape Bus/LConn12 -- Connection Label47/LConn1
  Simscape Bus/LConn11 -- Connection Label41/LConn1
  Simscape Bus/LConn10 -- Connection Label46/LConn1
  Simscape Bus/LConn9 -- Connection Label40/LConn1
  Simscape Bus/LConn8 -- Connection Label45/LConn1
  Simscape Bus/LConn7 -- Connection Label39/LConn1
  Simscape Bus/LConn6 -- Connection Label44/LConn1
  Simscape Bus/LConn5 -- Connection Label38/LConn1
  Simscape Bus/LConn4 -- Connection Label43/LConn1
  Simscape Bus/LConn3 -- Connection Label37/LConn1
  Simscape Bus/LConn2 -- Connection Label42/LConn1
  Simscape Bus/LConn1 -- Connection Label36/LConn1
  Connection Label48/LConn1 -- Rod 1/RConn2
  Connection Label54/LConn1 -- Rod 1/RConn4
  Rod 2/RConn2 -- Connection Label49/LConn1
  Connection Label55/LConn1 -- Rod 2/RConn4
  Connection Label50/LConn1 -- Rod 3/RConn2
  Connection Label56/LConn1 -- Rod 3/RConn4
  Connection Label51/LConn1 -- Rod 4/RConn2
  Connection Label57/LConn1 -- Rod 4/RConn4
  Connection Label52/LConn1 -- Rod 5/RConn2
  Connection Label58/LConn1 -- Rod 5/RConn4
  Connection Label53/LConn1 -- Rod 6/RConn2
  Connection Label59/LConn1 -- Rod 6/RConn4
  Connection Label28/LConn1 -- Simscape Bus1/LConn6

== system six_rod_tensegrity_model_2021a/Physical system/Rods/Rod 1 ==
  Center to right : sm_lib/Frames and Transforms/Rigid Transform  TranslationMethod=StandardAxis  TranslationStandardOffset=rod_end_offset  TranslationLengthUnit=m  TranslationStandardAxis=+Z  TranslationCartesianOffset=[0 400 0]  TranslationROffset=0  TranslationROffsetUnits=m  TranslationZOffset=0  TranslationZOffsetUnits=m  TranslationThetaOffset=0  TranslationThetaOffsetUnits=deg  RotationMethod=None  RotationAngleUnits=deg  RotationStandardAxis=+Y  RotationAngle=90  RotationArbitraryAxis=[0 0 1]  FollAlignAxisA=+Z  BaseAlignAxisA=+X  FollAlignAxisB=+Y  BaseAlignAxisB=+Z  RotationSequenceAxes=FollowerAxes  RotationSequence=XYX  RotationSequenceAngles=[0 0 0]  RotationSequenceAnglesUnits=deg  RotationMatrix=[1 0 0; 0 1 0; 0 0 1]
  Left end cap : sm_lib/Body Elements/Spherical Solid  GraphicAmbientColor=[0.15 0.15 0.15 1.0]  BasedOnType=Density  CenterOfMass=[0 0 0]  CenterOfMassUnits=m  GraphicDiffuseColor=rod_end_color  Density=1000  DensityUnits=kg/m^3  DoExposeReferenceFrame=on  GraphicEmissiveColor=[0.0 0.0 0.0 1.0]  ExportEntireGeometry=on  SerializedExposedGeometries=<ExposedGeometries><ExposedGeometry><RawGeometryId>entire</RawGeometryId><ExposedGeometryId>G</ExposedGeometryId></ExposedGeometry></ExposedGeometries>  SerializedFrames=<Frames/>  MarkerShape=Sphere  MarkerSize=10  GraphicType=FromGeometry  InertiaType=PointMass  Mass=rod_end_mass  MassUnits=kg  MomentsOfInertia=[1 1 1]  MomentsOfInertiaUnits=kg*m^2  GraphicOpacity=rod_end_opacity  ProductsOfInertia=[0 0 0]  ProductsOfInertiaUnits=kg*m^2  GraphicShininess=75  GraphicSpecularColor=[0.5 0.5 0.5 1.0]  SphereRadius=rod_end_radius  SphereRadiusUnits=m  GraphicVisPropType=SimpleVisualProperties
  Left to center : sm_lib/Frames and Transforms/Rigid Transform  TranslationMethod=StandardAxis  TranslationStandardOffset=rod_end_offset  TranslationLengthUnit=m  TranslationStandardAxis=+Z  TranslationCartesianOffset=[0 400 0]  TranslationROffset=0  TranslationROffsetUnits=m  TranslationZOffset=0  TranslationZOffsetUnits=m  TranslationThetaOffset=0  TranslationThetaOffsetUnits=deg  RotationMethod=None  RotationAngleUnits=deg  RotationStandardAxis=+Y  RotationAngle=90  RotationArbitraryAxis=[0 0 1]  FollAlignAxisA=+Z  BaseAlignAxisA=+X  FollAlignAxisB=+Y  BaseAlignAxisB=+Z  RotationSequenceAxes=FollowerAxes  RotationSequence=XYX  RotationSequenceAngles=[0 0 0]  RotationSequenceAnglesUnits=deg  RotationMatrix=[1 0 0; 0 1 0; 0 0 1]
  Right end cap : sm_lib/Body Elements/Spherical Solid  GraphicAmbientColor=[0.15 0.15 0.15 1.0]  BasedOnType=Density  CenterOfMass=[0 0 0]  CenterOfMassUnits=m  GraphicDiffuseColor=rod_end_color  Density=1000  DensityUnits=kg/m^3  DoExposeReferenceFrame=on  GraphicEmissiveColor=[0.0 0.0 0.0 1.0]  ExportEntireGeometry=on  SerializedExposedGeometries=<ExposedGeometries><ExposedGeometry><RawGeometryId>entire</RawGeometryId><ExposedGeometryId>G</ExposedGeometryId></ExposedGeometry></ExposedGeometries>  SerializedFrames=<Frames/>  MarkerShape=Sphere  MarkerSize=10  GraphicType=FromGeometry  InertiaType=PointMass  Mass=rod_end_mass  MassUnits=kg  MomentsOfInertia=[1 1 1]  MomentsOfInertiaUnits=kg*m^2  GraphicOpacity=rod_end_opacity  ProductsOfInertia=[0 0 0]  ProductsOfInertiaUnits=kg*m^2  GraphicShininess=75  GraphicSpecularColor=[0.5 0.5 0.5 1.0]  SphereRadius=rod_end_radius  SphereRadiusUnits=m  GraphicVisPropType=SimpleVisualProperties
  Rod : sm_lib/Body Elements/Revolved Solid  GraphicAmbientColor=[0.15 0.15 0.15 1.0]  BasedOnType=Mass  CenterOfMass=[0 0 0]  CenterOfMassUnits=m  GraphicDiffuseColor=rod_color  ExportConvexHullGeometry=off  Density=1000  DensityUnits=kg/m^3  DoExposeReferenceFrame=on  GraphicEmissiveColor=[0.0 0.0 0.0 1.0]  ExportEntireGeometry=off  SerializedFrames=<Frames/>  MarkerShape=Sphere  MarkerSize=10  GraphicType=FromGeometry  InertiaType=CalculateFromGeometry  Mass=rod_mass  MassUnits=kg  MomentsOfInertia=[1 1 1]  MomentsOfInertiaUnits=kg*m^2  GraphicOpacity=rod_opacity  ProductsOfInertia=[0 0 0]  ProductsOfInertiaUnits=kg*m^2  RevolutionCrossSection=rod_cross_section  RevolutionCrossSectionUnits=m  RevolutionAngle=180  RevolutionAngleUnits=deg  RevolutionExtent=Full  GraphicShininess=75  GraphicSpecularColor=[0.5 0.5 0.5 1.0]  GraphicVisPropType=SimpleVisualProperties
  to world : PMIOPort  Side=Left
  Left end cap [1] : PMIOPort  Port=2  Side=Right
  "Left end cap contact [1] " : PMIOPort  Port=3  Side=Right
  Right end cap [2] : PMIOPort  Port=4  Side=Right
  Right end cap contact [2] : PMIOPort  Port=5  Side=Right
  Rod center : PMIOPort  Port=6  Side=Right
  connections:
  Left to center/RConn1 -- Rod/RConn1 -- Rod center/RConn1 -- Center to right/LConn1
  to world/RConn1 -- Left end cap/RConn1 -- Left to center/LConn1 -- Left end cap [1]/RConn1
  Right end cap [2]/RConn1 -- Right end cap/RConn1 -- Center to right/RConn1
  Left end cap/LConn1 -- "Left end cap contact [1] "/RConn1
  Right end cap/LConn1 -- Right end cap contact [2]/RConn1

== system six_rod_tensegrity_model_2021a/Physical system/Rods/Rod 2 ==
  Center to right : sm_lib/Frames and Transforms/Rigid Transform  TranslationMethod=StandardAxis  TranslationStandardOffset=rod_end_offset_with_drive  TranslationLengthUnit=m  TranslationStandardAxis=+Z  TranslationCartesianOffset=[0 400 0]  TranslationROffset=0  TranslationROffsetUnits=m  TranslationZOffset=0  TranslationZOffsetUnits=m  TranslationThetaOffset=0  TranslationThetaOffsetUnits=deg  RotationMethod=None  RotationAngleUnits=deg  RotationStandardAxis=+Y  RotationAngle=90  RotationArbitraryAxis=[0 0 1]  FollAlignAxisA=+Z  BaseAlignAxisA=+X  FollAlignAxisB=+Y  BaseAlignAxisB=+Z  RotationSequenceAxes=FollowerAxes  RotationSequence=XYX  RotationSequenceAngles=[0 0 0]  RotationSequenceAnglesUnits=deg  RotationMatrix=[1 0 0; 0 1 0; 0 0 1]
  Left drive offset : sm_lib/Frames and Transforms/Rigid Transform  TranslationMethod=StandardAxis  TranslationStandardOffset=rod_end_drive_offset  TranslationLengthUnit=m  TranslationStandardAxis=+Z  TranslationCartesianOffset=[0 400 0]  TranslationROffset=0  TranslationROffsetUnits=m  TranslationZOffset=0  TranslationZOffsetUnits=m  TranslationThetaOffset=0  TranslationThetaOffsetUnits=deg  RotationMethod=None  RotationAngleUnits=deg  RotationStandardAxis=+Y  RotationAngle=90  RotationArbitraryAxis=[0 0 1]  FollAlignAxisA=+Z  BaseAlignAxisA=+X  FollAlignAxisB=+Y  BaseAlignAxisB=+Z  RotationSequenceAxes=FollowerAxes  RotationSequence=XYX  RotationSequenceAngles=[0 0 0]  RotationSequenceAnglesUnits=deg  RotationMatrix=[1 0 0; 0 1 0; 0 0 1]
  Left end cap : sm_lib/Body Elements/Spherical Solid  GraphicAmbientColor=[0.15 0.15 0.15 1.0]  BasedOnType=Density  CenterOfMass=[0 0 0]  CenterOfMassUnits=m  GraphicDiffuseColor=rod_end_color_with_drive  Density=1000  DensityUnits=kg/m^3  DoExposeReferenceFrame=on  GraphicEmissiveColor=[0.0 0.0 0.0 1.0]  ExportEntireGeometry=on  SerializedExposedGeometries=<ExposedGeometries><ExposedGeometry><RawGeometryId>entire</RawGeometryId><ExposedGeometryId>G</ExposedGeometryId></ExposedGeometry></ExposedGeometries>  SerializedFrames=<Frames/>  MarkerShape=Sphere  MarkerSize=10  GraphicType=FromGeometry  InertiaType=PointMass  Mass=rod_end_mass_with_drive  MassUnits=kg  MomentsOfInertia=[1 1 1]  MomentsOfInertiaUnits=kg*m^2  GraphicOpacity=rod_end_opacity_with_drive  ProductsOfInertia=[0 0 0]  ProductsOfInertiaUnits=kg*m^2  GraphicShininess=75  GraphicSpecularColor=[0.5 0.5 0.5 1.0]  SphereRadius=rod_end_radius  SphereRadiusUnits=m  GraphicVisPropType=SimpleVisualProperties
  Left to center : sm_lib/Frames and Transforms/Rigid Transform  TranslationMethod=StandardAxis  TranslationStandardOffset=rod_end_offset_with_drive  TranslationLengthUnit=m  TranslationStandardAxis=+Z  TranslationCartesianOffset=[0 400 0]  TranslationROffset=0  TranslationROffsetUnits=m  TranslationZOffset=0  TranslationZOffsetUnits=m  TranslationThetaOffset=0  TranslationThetaOffsetUnits=deg  RotationMethod=None  RotationAngleUnits=deg  RotationStandardAxis=+Y  RotationAngle=90  RotationArbitraryAxis=[0 0 1]  FollAlignAxisA=+Z  BaseAlignAxisA=+X  FollAlignAxisB=+Y  BaseAlignAxisB=+Z  RotationSequenceAxes=FollowerAxes  RotationSequence=XYX  RotationSequenceAngles=[0 0 0]  RotationSequenceAnglesUnits=deg  RotationMatrix=[1 0 0; 0 1 0; 0 0 1]
  Right drive offset : sm_lib/Frames and Transforms/Rigid Transform  TranslationMethod=StandardAxis  TranslationStandardOffset=rod_end_drive_offset  TranslationLengthUnit=m  TranslationStandardAxis=+Z  TranslationCartesianOffset=[0 400 0]  TranslationROffset=0  TranslationROffsetUnits=m  TranslationZOffset=0  TranslationZOffsetUnits=m  TranslationThetaOffset=0  TranslationThetaOffsetUnits=deg  RotationMethod=None  RotationAngleUnits=deg  RotationStandardAxis=+Y  RotationAngle=90  RotationArbitraryAxis=[0 0 1]  FollAlignAxisA=+Z  BaseAlignAxisA=+X  FollAlignAxisB=+Y  BaseAlignAxisB=+Z  RotationSequenceAxes=FollowerAxes  RotationSequence=XYX  RotationSequenceAngles=[0 0 0]  RotationSequenceAnglesUnits=deg  RotationMatrix=[1 0 0; 0 1 0; 0 0 1]
  Right end cap : sm_lib/Body Elements/Spherical Solid  GraphicAmbientColor=[0.15 0.15 0.15 1.0]  BasedOnType=Density  CenterOfMass=[0 0 0]  CenterOfMassUnits=m  GraphicDiffuseColor=rod_end_color_with_drive  Density=1000  DensityUnits=kg/m^3  DoExposeReferenceFrame=on  GraphicEmissiveColor=[0.0 0.0 0.0 1.0]  ExportEntireGeometry=on  SerializedExposedGeometries=<ExposedGeometries><ExposedGeometry><RawGeometryId>entire</RawGeometryId><ExposedGeometryId>G</ExposedGeometryId></ExposedGeometry></ExposedGeometries>  SerializedFrames=<Frames/>  MarkerShape=Sphere  MarkerSize=10  GraphicType=FromGeometry  InertiaType=PointMass  Mass=rod_end_mass_with_drive  MassUnits=kg  MomentsOfInertia=[1 1 1]  MomentsOfInertiaUnits=kg*m^2  GraphicOpacity=rod_end_opacity_with_drive  ProductsOfInertia=[0 0 0]  ProductsOfInertiaUnits=kg*m^2  GraphicShininess=75  GraphicSpecularColor=[0.5 0.5 0.5 1.0]  SphereRadius=rod_end_radius  SphereRadiusUnits=m  GraphicVisPropType=SimpleVisualProperties
  Rod : sm_lib/Body Elements/Revolved Solid  GraphicAmbientColor=[0.15 0.15 0.15 1.0]  BasedOnType=Mass  CenterOfMass=[0 0 0]  CenterOfMassUnits=m  GraphicDiffuseColor=rod_color_with_drive  ExportConvexHullGeometry=off  Density=1000  DensityUnits=kg/m^3  DoExposeReferenceFrame=on  GraphicEmissiveColor=[0.0 0.0 0.0 1.0]  ExportEntireGeometry=off  SerializedFrames=<Frames/>  MarkerShape=Sphere  MarkerSize=10  GraphicType=FromGeometry  InertiaType=CalculateFromGeometry  Mass=rod_mass_with_drive  MassUnits=kg  MomentsOfInertia=[1 1 1]  MomentsOfInertiaUnits=kg*m^2  GraphicOpacity=rod_opacity_with_drive  ProductsOfInertia=[0 0 0]  ProductsOfInertiaUnits=kg*m^2  RevolutionCrossSection=rod_cross_section_with_drive  RevolutionCrossSectionUnits=m  RevolutionAngle=180  RevolutionAngleUnits=deg  RevolutionExtent=Full  GraphicShininess=75  GraphicSpecularColor=[0.5 0.5 0.5 1.0]  GraphicVisPropType=SimpleVisualProperties
  to world : PMIOPort  Side=Left
  Left end cap [3] : PMIOPort  Port=2  Side=Right
  "Left end cap contact [3] " : PMIOPort  Port=3  Side=Right
  Right end cap [4] : PMIOPort  Port=4  Side=Right
  Right end cap contact [4] : PMIOPort  Port=5  Side=Right
  Rod center : PMIOPort  Port=6  Side=Right
  connections:
  Right end cap/RConn1 -- Right drive offset/RConn1
  Rod/RConn1 -- Left to center/RConn1 -- Center to right/LConn1 -- Rod center/RConn1
  to world/RConn1 -- Left end cap/RConn1 -- Left drive offset/LConn1
  "Left end cap contact [3] "/RConn1 -- Left end cap/LConn1
  Right end cap contact [4]/RConn1 -- Right end cap/LConn1
  Left drive offset/RConn1 -- Left end cap [3]/RConn1 -- Left to center/LConn1
  Right drive offset/LConn1 -- Right end cap [4]/RConn1 -- Center to right/RConn1

== system six_rod_tensegrity_model_2021a/Physical system/Rods/Rod 3 ==
  Center to right : sm_lib/Frames and Transforms/Rigid Transform  TranslationMethod=StandardAxis  TranslationStandardOffset=rod_end_offset_with_drive  TranslationLengthUnit=m  TranslationStandardAxis=+Z  TranslationCartesianOffset=[0 400 0]  TranslationROffset=0  TranslationROffsetUnits=m  TranslationZOffset=0  TranslationZOffsetUnits=m  TranslationThetaOffset=0  TranslationThetaOffsetUnits=deg  RotationMethod=None  RotationAngleUnits=deg  RotationStandardAxis=+Y  RotationAngle=90  RotationArbitraryAxis=[0 0 1]  FollAlignAxisA=+Z  BaseAlignAxisA=+X  FollAlignAxisB=+Y  BaseAlignAxisB=+Z  RotationSequenceAxes=FollowerAxes  RotationSequence=XYX  RotationSequenceAngles=[0 0 0]  RotationSequenceAnglesUnits=deg  RotationMatrix=[1 0 0; 0 1 0; 0 0 1]
  Left drive offset : sm_lib/Frames and Transforms/Rigid Transform  TranslationMethod=StandardAxis  TranslationStandardOffset=rod_end_drive_offset  TranslationLengthUnit=m  TranslationStandardAxis=+Z  TranslationCartesianOffset=[0 400 0]  TranslationROffset=0  TranslationROffsetUnits=m  TranslationZOffset=0  TranslationZOffsetUnits=m  TranslationThetaOffset=0  TranslationThetaOffsetUnits=deg  RotationMethod=None  RotationAngleUnits=deg  RotationStandardAxis=+Y  RotationAngle=90  RotationArbitraryAxis=[0 0 1]  FollAlignAxisA=+Z  BaseAlignAxisA=+X  FollAlignAxisB=+Y  BaseAlignAxisB=+Z  RotationSequenceAxes=FollowerAxes  RotationSequence=XYX  RotationSequenceAngles=[0 0 0]  RotationSequenceAnglesUnits=deg  RotationMatrix=[1 0 0; 0 1 0; 0 0 1]
  Left end cap : sm_lib/Body Elements/Spherical Solid  GraphicAmbientColor=[0.15 0.15 0.15 1.0]  BasedOnType=Density  CenterOfMass=[0 0 0]  CenterOfMassUnits=m  GraphicDiffuseColor=rod_end_color_with_drive  Density=1000  DensityUnits=kg/m^3  DoExposeReferenceFrame=on  GraphicEmissiveColor=[0.0 0.0 0.0 1.0]  ExportEntireGeometry=on  SerializedExposedGeometries=<ExposedGeometries><ExposedGeometry><RawGeometryId>entire</RawGeometryId><ExposedGeometryId>G</ExposedGeometryId></ExposedGeometry></ExposedGeometries>  SerializedFrames=<Frames/>  MarkerShape=Sphere  MarkerSize=10  GraphicType=FromGeometry  InertiaType=PointMass  Mass=rod_end_mass_with_drive  MassUnits=kg  MomentsOfInertia=[1 1 1]  MomentsOfInertiaUnits=kg*m^2  GraphicOpacity=rod_end_opacity_with_drive  ProductsOfInertia=[0 0 0]  ProductsOfInertiaUnits=kg*m^2  GraphicShininess=75  GraphicSpecularColor=[0.5 0.5 0.5 1.0]  SphereRadius=rod_end_radius  SphereRadiusUnits=m  GraphicVisPropType=SimpleVisualProperties
  Left to center : sm_lib/Frames and Transforms/Rigid Transform  TranslationMethod=StandardAxis  TranslationStandardOffset=rod_end_offset_with_drive  TranslationLengthUnit=m  TranslationStandardAxis=+Z  TranslationCartesianOffset=[0 400 0]  TranslationROffset=0  TranslationROffsetUnits=m  TranslationZOffset=0  TranslationZOffsetUnits=m  TranslationThetaOffset=0  TranslationThetaOffsetUnits=deg  RotationMethod=None  RotationAngleUnits=deg  RotationStandardAxis=+Y  RotationAngle=90  RotationArbitraryAxis=[0 0 1]  FollAlignAxisA=+Z  BaseAlignAxisA=+X  FollAlignAxisB=+Y  BaseAlignAxisB=+Z  RotationSequenceAxes=FollowerAxes  RotationSequence=XYX  RotationSequenceAngles=[0 0 0]  RotationSequenceAnglesUnits=deg  RotationMatrix=[1 0 0; 0 1 0; 0 0 1]
  Right drive offset : sm_lib/Frames and Transforms/Rigid Transform  TranslationMethod=StandardAxis  TranslationStandardOffset=rod_end_drive_offset  TranslationLengthUnit=m  TranslationStandardAxis=+Z  TranslationCartesianOffset=[0 400 0]  TranslationROffset=0  TranslationROffsetUnits=m  TranslationZOffset=0  TranslationZOffsetUnits=m  TranslationThetaOffset=0  TranslationThetaOffsetUnits=deg  RotationMethod=None  RotationAngleUnits=deg  RotationStandardAxis=+Y  RotationAngle=90  RotationArbitraryAxis=[0 0 1]  FollAlignAxisA=+Z  BaseAlignAxisA=+X  FollAlignAxisB=+Y  BaseAlignAxisB=+Z  RotationSequenceAxes=FollowerAxes  RotationSequence=XYX  RotationSequenceAngles=[0 0 0]  RotationSequenceAnglesUnits=deg  RotationMatrix=[1 0 0; 0 1 0; 0 0 1]
  Right end cap : sm_lib/Body Elements/Spherical Solid  GraphicAmbientColor=[0.15 0.15 0.15 1.0]  BasedOnType=Density  CenterOfMass=[0 0 0]  CenterOfMassUnits=m  GraphicDiffuseColor=rod_end_color_with_drive  Density=1000  DensityUnits=kg/m^3  DoExposeReferenceFrame=on  GraphicEmissiveColor=[0.0 0.0 0.0 1.0]  ExportEntireGeometry=on  SerializedExposedGeometries=<ExposedGeometries><ExposedGeometry><RawGeometryId>entire</RawGeometryId><ExposedGeometryId>G</ExposedGeometryId></ExposedGeometry></ExposedGeometries>  SerializedFrames=<Frames/>  MarkerShape=Sphere  MarkerSize=10  GraphicType=FromGeometry  InertiaType=PointMass  Mass=rod_end_mass_with_drive  MassUnits=kg  MomentsOfInertia=[1 1 1]  MomentsOfInertiaUnits=kg*m^2  GraphicOpacity=rod_end_opacity_with_drive  ProductsOfInertia=[0 0 0]  ProductsOfInertiaUnits=kg*m^2  GraphicShininess=75  GraphicSpecularColor=[0.5 0.5 0.5 1.0]  SphereRadius=rod_end_radius  SphereRadiusUnits=m  GraphicVisPropType=SimpleVisualProperties
  Rod : sm_lib/Body Elements/Revolved Solid  GraphicAmbientColor=[0.15 0.15 0.15 1.0]  BasedOnType=Mass  CenterOfMass=[0 0 0]  CenterOfMassUnits=m  GraphicDiffuseColor=rod_color_with_drive  ExportConvexHullGeometry=off  Density=1000  DensityUnits=kg/m^3  DoExposeReferenceFrame=on  GraphicEmissiveColor=[0.0 0.0 0.0 1.0]  ExportEntireGeometry=off  SerializedFrames=<Frames/>  MarkerShape=Sphere  MarkerSize=10  GraphicType=FromGeometry  InertiaType=CalculateFromGeometry  Mass=rod_mass_with_drive  MassUnits=kg  MomentsOfInertia=[1 1 1]  MomentsOfInertiaUnits=kg*m^2  GraphicOpacity=rod_opacity_with_drive  ProductsOfInertia=[0 0 0]  ProductsOfInertiaUnits=kg*m^2  RevolutionCrossSection=rod_cross_section_with_drive  RevolutionCrossSectionUnits=m  RevolutionAngle=180  RevolutionAngleUnits=deg  RevolutionExtent=Full  GraphicShininess=75  GraphicSpecularColor=[0.5 0.5 0.5 1.0]  GraphicVisPropType=SimpleVisualProperties
  to world : PMIOPort  Side=Left
  Left end cap [5] : PMIOPort  Port=2  Side=Right
  "Left end cap contact [5] " : PMIOPort  Port=3  Side=Right
  Right end cap [6] : PMIOPort  Port=4  Side=Right
  Right end cap contact [6] : PMIOPort  Port=5  Side=Right
  Rod center : PMIOPort  Port=6  Side=Right
  connections:
  Rod center/RConn1 -- Center to right/LConn1 -- Left to center/RConn1 -- Rod/RConn1
  Left end cap/RConn1 -- Left drive offset/LConn1 -- to world/RConn1
  Left end cap/LConn1 -- "Left end cap contact [5] "/RConn1
  Right end cap/LConn1 -- Right end cap contact [6]/RConn1
  Left drive offset/RConn1 -- Left end cap [5]/RConn1 -- Left to center/LConn1
  Right end cap/RConn1 -- Right drive offset/RConn1
  Center to right/RConn1 -- Right end cap [6]/RConn1 -- Right drive offset/LConn1
